simulink model "cyberAttack2"  (R2022b)
settings: Solver=VariableStepAuto  StartTime=0.0  StopTime=10  RelTol=1e-3
values from neighbouring files (symbols this model uses):
  attackTimeDelay = 0.1    [editor.m]
  attackTimeDelay1 = 0.1    [editor.m]
  CC_Kd = 0    [editor.m]
  CC_Ki = 150    [editor.m]
  CC_Kp = 0    [editor.m]
  enableObserver = 1    [editor.m]
  ICapacity_1 = 3    [editor.m]
  ICapacity_2 = 2    [editor.m]
  ILoadFinal = 2    [editor.m]
  ILoadInitial = 3    [editor.m]
  Kd = 4.6e-4    (= 0.00046)    [editor.m]
  Ki = 6.15    [editor.m]
  Kp = 0.1    [editor.m]
  N = 2.56e3    (= 2560)    [editor.m]
  Rij = 0.05    [editor.m]
  Rt = 0.2    [editor.m]
  timeOfAttack = 5    [editor.m]
  timeOfAttack1 = 5    [editor.m]
  tLoadChange = 6    [editor.m]
  Ts = 5e-5    (= 5e-05)    [editor.m]
  Vref = 40    [editor.m]
undefined symbols (not defined in the file or in its folder): Discrete, Time
libraries: fl_lib x54, nesl_utility_internal x30, slpidlib x8, simulink x4, ctrlSharedLib x4, ee_lib x4
(part 2 of 3)

== system cyberAttack2/DGU 1 Observer1 ==
  Vout_3_local : Inport
  It_3_local : Inport  Port=2
  Vt_3 : Inport  Port=3
  Vout_3 : Inport  Port=4
  Vout_4 : Inport  Port=5
  IL : Inport  Port=6
  Disabled : Subsystem  VariantControl=enableObserver == 0
      settings: PortSchema="{\"entries\":[{\"content\":{\"sides\":[{\"content\":{\"connectorIds\":[\"In1\",\"In2\",\"In3\",\"In4\"]},\"type\":\"ConnectorPlacement.EquallySpacedRectSide\",\"uuid\":\"1fcbc3c4-c380-448d-a7a8-357aa057b5ad\"},{\"content\":{\"connectorIds\":[\"Out1\",\"Out2\",\"Out3\"],\"side\":\"RIGHT\"},\"type\":\"ConnectorPlacement.EquallySpacedRectSide\",\"uuid\":\"7cbaad62-7890-4094-8ace-3159eca04825\"},{\"content\":{\"connectorIds\":[\"In5\",\"In6\"],\"side\":\"TOP\"},\"type\":\"ConnectorPlacement.EquallySpacedRectSide\",\"uuid\":\"f6c34017-9df2-4479-96e0-d67eb53c1d2d\"}]},\"type\":\"ConnectorPlacement.EquallySpacedConnector\",\"uuid\":\"f0a4a9b8-ed06-4c65-915f-6b202d377626\"}],\"packageUris\":[\"http://schema.mathworks.com/mf0/Connector/R2020b\"],\"version\":\"1.0\"}"
  Enabled : Subsystem  VariantControl=enableObserver == 1
      settings: PortSchema="{\"entries\":[{\"content\":{\"sides\":[{\"content\":{\"connectorIds\":[\"In1\",\"In2\",\"In3\",\"In4\"]},\"type\":\"ConnectorPlacement.EquallySpacedRectSide\",\"uuid\":\"1fcbc3c4-c380-448d-a7a8-357aa057b5ad\"},{\"content\":{\"connectorIds\":[\"Out1\",\"Out2\",\"Out3\"],\"side\":\"RIGHT\"},\"type\":\"ConnectorPlacement.EquallySpacedRectSide\",\"uuid\":\"7cbaad62-7890-4094-8ace-3159eca04825\"},{\"content\":{\"connectorIds\":[\"In5\",\"In6\"],\"side\":\"TOP\"},\"type\":\"ConnectorPlacement.EquallySpacedRectSide\",\"uuid\":\"f6c34017-9df2-4479-96e0-d67eb53c1d2d\"}]},\"type\":\"ConnectorPlacement.EquallySpacedConnector\",\"uuid\":\"f0a4a9b8-ed06-4c65-915f-6b202d377626\"}],\"packageUris\":[\"http://schema.mathworks.com/mf0/Connector/R2020b\"],\"version\":\"1.0\"}"
  residual_Vout : Outport
  residual_It : Outport  Port=2
  attackDetected : Outport  Port=3

== system cyberAttack2/DGU 2 Observer ==
  Vout_2_local : Inport
  It_2_local : Inport  Port=2
  Vt_2 : Inport  Port=3
  Vout_2 : Inport  Port=4
  Vout_1 : Inport  Port=5
  IL : Inport  Port=6
  Disabled : Subsystem  VariantControl=enableObserver == 0
      settings: PortSchema="{\"entries\":[{\"content\":{\"sides\":[{\"content\":{\"connectorIds\":[\"In1\",\"In2\",\"In3\",\"In4\"]},\"type\":\"ConnectorPlacement.EquallySpacedRectSide\",\"uuid\":\"1fcbc3c4-c380-448d-a7a8-357aa057b5ad\"},{\"content\":{\"connectorIds\":[\"Out1\",\"Out2\",\"Out3\"],\"side\":\"RIGHT\"},\"type\":\"ConnectorPlacement.EquallySpacedRectSide\",\"uuid\":\"7cbaad62-7890-4094-8ace-3159eca04825\"},{\"content\":{\"connectorIds\":[\"In5\",\"In6\"],\"side\":\"TOP\"},\"type\":\"ConnectorPlacement.EquallySpacedRectSide\",\"uuid\":\"f6c34017-9df2-4479-96e0-d67eb53c1d2d\"}]},\"type\":\"ConnectorPlacement.EquallySpacedConnector\",\"uuid\":\"f0a4a9b8-ed06-4c65-915f-6b202d377626\"}],\"packageUris\":[\"http://schema.mathworks.com/mf0/Connector/R2020b\"],\"version\":\"1.0\"}"
  Enabled : Subsystem  VariantControl=enableObserver == 1
      settings: PortSchema="{\"entries\":[{\"content\":{\"sides\":[{\"content\":{\"connectorIds\":[\"In1\",\"In2\",\"In3\",\"In4\"]},\"type\":\"ConnectorPlacement.EquallySpacedRectSide\",\"uuid\":\"1fcbc3c4-c380-448d-a7a8-357aa057b5ad\"},{\"content\":{\"connectorIds\":[\"Out1\",\"Out2\",\"Out3\"],\"side\":\"RIGHT\"},\"type\":\"ConnectorPlacement.EquallySpacedRectSide\",\"uuid\":\"7cbaad62-7890-4094-8ace-3159eca04825\"},{\"content\":{\"connectorIds\":[\"In5\",\"In6\"],\"side\":\"TOP\"},\"type\":\"ConnectorPlacement.EquallySpacedRectSide\",\"uuid\":\"f6c34017-9df2-4479-96e0-d67eb53c1d2d\"}]},\"type\":\"ConnectorPlacement.EquallySpacedConnector\",\"uuid\":\"f0a4a9b8-ed06-4c65-915f-6b202d377626\"}],\"packageUris\":[\"http://schema.mathworks.com/mf0/Connector/R2020b\"],\"version\":\"1.0\"}"
  residual_Vout : Outport
  residual_It : Outport  Port=2
  attackDetected : Outport  Port=3

== system cyberAttack2/DGU 2 Observer1 ==
  Vout_4_local : Inport
  It_4_local : Inport  Port=2
  Vt_4 : Inport  Port=3
  Vout_4 : Inport  Port=4
  Vout_3 : Inport  Port=5
  IL : Inport  Port=6
  Disabled : Subsystem  VariantControl=enableObserver == 0
      settings: PortSchema="{\"entries\":[{\"content\":{\"sides\":[{\"content\":{\"connectorIds\":[\"In1\",\"In2\",\"In3\",\"In4\"]},\"type\":\"ConnectorPlacement.EquallySpacedRectSide\",\"uuid\":\"1fcbc3c4-c380-448d-a7a8-357aa057b5ad\"},{\"content\":{\"connectorIds\":[\"Out1\",\"Out2\",\"Out3\"],\"side\":\"RIGHT\"},\"type\":\"ConnectorPlacement.EquallySpacedRectSide\",\"uuid\":\"7cbaad62-7890-4094-8ace-3159eca04825\"},{\"content\":{\"connectorIds\":[\"In5\",\"In6\"],\"side\":\"TOP\"},\"type\":\"ConnectorPlacement.EquallySpacedRectSide\",\"uuid\":\"f6c34017-9df2-4479-96e0-d67eb53c1d2d\"}]},\"type\":\"ConnectorPlacement.EquallySpacedConnector\",\"uuid\":\"f0a4a9b8-ed06-4c65-915f-6b202d377626\"}],\"packageUris\":[\"http://schema.mathworks.com/mf0/Connector/R2020b\"],\"version\":\"1.0\"}"
  Enabled : Subsystem  VariantControl=enableObserver == 1
      settings: PortSchema="{\"entries\":[{\"content\":{\"sides\":[{\"content\":{\"connectorIds\":[\"In1\",\"In2\",\"In3\",\"In4\"]},\"type\":\"ConnectorPlacement.EquallySpacedRectSide\",\"uuid\":\"1fcbc3c4-c380-448d-a7a8-357aa057b5ad\"},{\"content\":{\"connectorIds\":[\"Out1\",\"Out2\",\"Out3\"],\"side\":\"RIGHT\"},\"type\":\"ConnectorPlacement.EquallySpacedRectSide\",\"uuid\":\"7cbaad62-7890-4094-8ace-3159eca04825\"},{\"content\":{\"connectorIds\":[\"In5\",\"In6\"],\"side\":\"TOP\"},\"type\":\"ConnectorPlacement.EquallySpacedRectSide\",\"uuid\":\"f6c34017-9df2-4479-96e0-d67eb53c1d2d\"}]},\"type\":\"ConnectorPlacement.EquallySpacedConnector\",\"uuid\":\"f0a4a9b8-ed06-4c65-915f-6b202d377626\"}],\"packageUris\":[\"http://schema.mathworks.com/mf0/Connector/R2020b\"],\"version\":\"1.0\"}"
  residual_Vout : Outport
  residual_It : Outport  Port=2
  attackDetected : Outport  Port=3

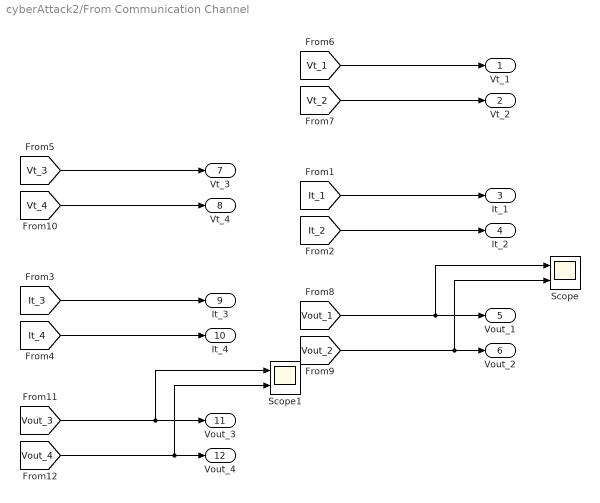
== system cyberAttack2/From Communication Channel ==
  Scope : Scope  NumInputPorts=2
  Scope1 : Scope  NumInputPorts=2
  Vt_1 : Outport
  Vt_2 : Outport  Port=2
  It_1 : Outport  Port=3
  It_2 : Outport  Port=4
  Vout_1 : Outport  Port=5
  Vout_2 : Outport  Port=6
  Vt_3 : Outport  Port=7
  Vt_4 : Outport  Port=8
  It_3 : Outport  Port=9
  It_4 : Outport  Port=10
  Vout_3 : Outport  Port=11
  Vout_4 : Outport  Port=12
  wires:
  [Vout_2] -> Scope/2, Vout_2/1
  [Vt_1] -> Vt_1/1
  [It_1] -> It_1/1
  [Vout_1] -> Scope/1, Vout_1/1
  [Vt_2] -> Vt_2/1
  [It_2] -> It_2/1
  [Vout_4] -> Scope1/2, Vout_4/1
  [Vout_3] -> Scope1/1, Vout_3/1
  [Vt_3] -> Vt_3/1
  [Vt_4] -> Vt_4/1
  [It_3] -> It_3/1
  [It_4] -> It_4/1

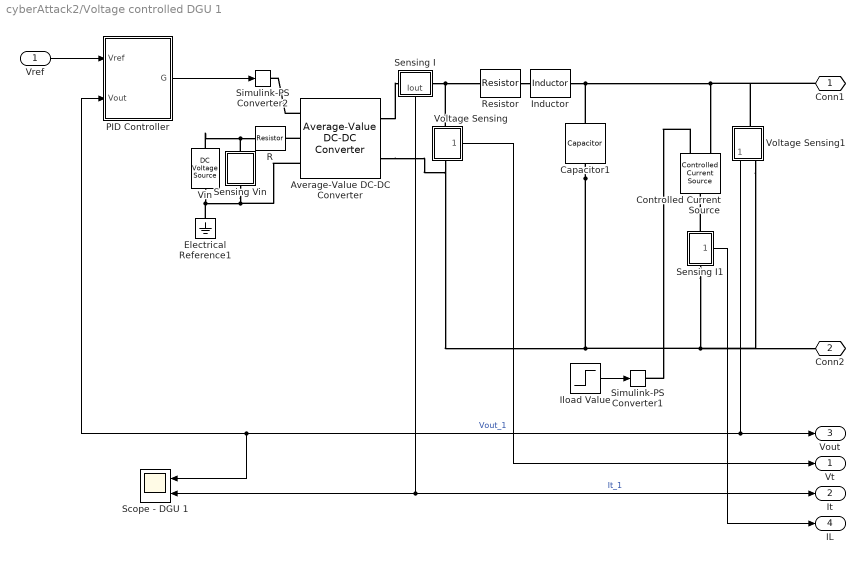
== system cyberAttack2/Voltage controlled DGU 1 ==
  Vref : Inport
  Average-Value DC-DC Converter : ee_lib/Semiconductors & Converters/Converters/Average-Value DC-DC Converter  control_option=ee.enum.converters.controlinput.dutycycle  converter_type=ee.enum.converters.dcdctype.buck  efficiency_option=ee.enum.converters.efficiency.constant  efficiency_fixed=100  i_vec=[0, 2, 5] A  efficiency_vec=[90, 95, 98]
      settings: InternalSimscapePortConfiguration="{\"Bottom\":[],\"Left\":[{\"id\":\"DutyCycle\",\"label\":\"DutyCycle\",\"type\":\"input\"},{\"id\":\"p1\",\"label\":\"1+\",\"type\":\"foundation.electrical.electrical\"},{\"id\":\"n1\",\"label\":\"1-\",\"type\":\"foundation.electrical.electrical\"}],\"Right\":[{\"id\":\"p2\",\"label\":\"2+\",\"type\":\"foundation.electrical.electrical\"},{\"id\":\"n2\",\"label\":\"2-\",\"type\":\"foundation.electrical.electrical\"}],\"Top\":[]}"
  Capacitor1 : fl_lib/Electrical/Electrical Elements/Capacitor  c=Ct F  r=1e-6 Ohm  g=0 1/Ohm  i_specify=off  i_priority=None  i=0 A  i_nominal_specify=off  i_nominal_unit=A  i_nominal_value=1  v_specify=on  v_priority=None  v=80 V  v_nominal_specify=off  v_nominal_unit=V  v_nominal_value=1  vc_specify=off  vc_priority=High  vc=0 V  vc_nominal_specify=off  vc_nominal_unit=V  vc_nominal_value=1
  Controlled Current Source : fl_lib/Electrical/Electrical Sources/Controlled Current Source
  Electrical Reference1 : fl_lib/Electrical/Electrical Elements/Electrical Reference
  Iload Value : Step  Time=tLoadChange  Before=ILoadInitial  After=ILoadFinal  SampleTime=Ts  VectorParams1D=off
  Inductor : fl_lib/Electrical/Electrical Elements/Inductor  l=Lt H  r=0 Ohm  g=1e-9 1/Ohm  i_specify=off  i_priority=None  i=0 A  i_nominal_specify=off  i_nominal_unit=A  i_nominal_value=1  v_specify=off  v_priority=None  v=0 V  v_nominal_specify=off  v_nominal_unit=V  v_nominal_value=1  i_L_specify=off  i_L_priority=High  i_L=0 A  i_L_nominal_specify=off  i_L_nominal_unit=A  i_L_nominal_value=1
  PID Controller : Subsystem  VariantControl=PID Controller
  R : fl_lib/Electrical/Electrical Elements/Resistor  R=0.001 Ohm  i_specify=off  i_priority=None  i=0 A  i_nominal_specify=off  i_nominal_unit=A  i_nominal_value=1  v_specify=off  v_priority=None  v=0 V  v_nominal_specify=off  v_nominal_unit=V  v_nominal_value=1
  Resistor : fl_lib/Electrical/Electrical Elements/Resistor  R=Rt Ohm  i_specify=off  i_priority=None  i=0 A  i_nominal_specify=off  i_nominal_unit=A  i_nominal_value=1  v_specify=off  v_priority=None  v=0 V  v_nominal_specify=off  v_nominal_unit=V  v_nominal_value=1
  Scope - DGU 1 : Scope  NumInputPorts=2
  Sensing Vin : Subsystem
      mask Display:
      | disp('V')
      | port_label('Lconn',1,'+')
      | port_label('Rconn',1,'-')
  Sensing I : Subsystem
      settings: PortSchema="{\"entries\":[{\"content\":{\"sides\":[{\"content\":{\"connectorIds\":[\"LConn1\"]},\"type\":\"ConnectorPlacement.EquallySpacedRectSide\",\"uuid\":\"8998040f-d19b-40f6-852f-9dc0afd5a871\"},{\"content\":{\"connectorIds\":[\"RConn1\"],\"side\":\"RIGHT\"},\"type\":\"ConnectorPlacement.EquallySpacedRectSide\",\"uuid\":\"65494d6e-d653-4050-90f0-55ab431a5ea5\"},{\"content\":{\"connectorIds\":[],\"side\":\"TOP\"},\"type\":\"ConnectorPlacement.EquallySpacedRectSide\",\"uuid\":\"2b796c8d-afa9-4f67-a302-9fd74e5c5a87\"},{\"content\":{\"connectorIds\":[\"Out1\"],\"side\":\"BOTTOM\"},\"type\":\"ConnectorPlacement.EquallySpacedRectSide\",\"uuid\":\"a59db07b-fad7-4423-9f0d-248c8e243318\"}]},\"type\":\"ConnectorPlacement.EquallySpacedConnector\",\"uuid\":\"55bdfac7-fde1-4547-95b0-f675ec2b07db\"}],\"packageUris\":[\"http://schema.mathworks.com/mf0/Connector/R2020b\"],\"version\":\"1.0\"}"
      mask Display:
      | disp('I')
      | port_label('Lconn',1,'+')
      | port_label('Rconn',1,'-')
  Sensing I1 : Subsystem
      settings: PortSchema="{\"entries\":[{\"content\":{\"sides\":[{\"content\":{\"connectorIds\":[\"LConn1\"]},\"type\":\"ConnectorPlacement.EquallySpacedRectSide\",\"uuid\":\"8998040f-d19b-40f6-852f-9dc0afd5a871\"},{\"content\":{\"connectorIds\":[\"RConn1\"],\"side\":\"RIGHT\"},\"type\":\"ConnectorPlacement.EquallySpacedRectSide\",\"uuid\":\"65494d6e-d653-4050-90f0-55ab431a5ea5\"},{\"content\":{\"connectorIds\":[\"Out1\"],\"side\":\"TOP\"},\"type\":\"ConnectorPlacement.EquallySpacedRectSide\",\"uuid\":\"2b796c8d-afa9-4f67-a302-9fd74e5c5a87\"},{\"content\":{\"connectorIds\":[],\"side\":\"BOTTOM\"},\"type\":\"ConnectorPlacement.EquallySpacedRectSide\",\"uuid\":\"a59db07b-fad7-4423-9f0d-248c8e243318\"}]},\"type\":\"ConnectorPlacement.EquallySpacedConnector\",\"uuid\":\"55bdfac7-fde1-4547-95b0-f675ec2b07db\"}],\"packageUris\":[\"http://schema.mathworks.com/mf0/Connector/R2020b\"],\"version\":\"1.0\"}"
      mask Display:
      | disp('I')
      | port_label('Lconn',1,'+')
      | port_label('Rconn',1,'-')
  Simulink-PS Converter1 : nesl_utility_internal/Simulink-PS Converter  PhysicalDomain=network_engine_domain  SubClassName=ps_input  LeftPortType=input  RightPortType=output  PseudoPeriodic=off  Frequencies=[]  NoiseDistribution=none  NoiseParameters=[]  Unit=1  AffineConversion=off  FilteringAndDerivatives=zero  SimscapeFilterOrder=1  InputFilterTimeConstant=0.001  UdotUserProvided=0
  Simulink-PS Converter2 : nesl_utility_internal/Simulink-PS Converter  PhysicalDomain=network_engine_domain  SubClassName=ps_input  LeftPortType=input  RightPortType=output  PseudoPeriodic=off  Frequencies=[]  NoiseDistribution=none  NoiseParameters=[]  Unit=1  AffineConversion=off  FilteringAndDerivatives=provide  SimscapeFilterOrder=1  InputFilterTimeConstant=0.001  UdotUserProvided=0
  Vin : fl_lib/Electrical/Electrical Sources/DC Voltage Source  v0=Vin V
  Voltage Sensing : Subsystem
      settings: PortSchema="{\"entries\":[{\"content\":{\"sides\":[{\"content\":{\"connectorIds\":[\"LConn1\"]},\"type\":\"ConnectorPlacement.EquallySpacedRectSide\",\"uuid\":\"8998040f-d19b-40f6-852f-9dc0afd5a871\"},{\"content\":{\"connectorIds\":[\"RConn1\"],\"side\":\"RIGHT\"},\"type\":\"ConnectorPlacement.EquallySpacedRectSide\",\"uuid\":\"65494d6e-d653-4050-90f0-55ab431a5ea5\"},{\"content\":{\"connectorIds\":[],\"side\":\"TOP\"},\"type\":\"ConnectorPlacement.EquallySpacedRectSide\",\"uuid\":\"2b796c8d-afa9-4f67-a302-9fd74e5c5a87\"},{\"content\":{\"connectorIds\":[\"Out1\"],\"side\":\"BOTTOM\"},\"type\":\"ConnectorPlacement.EquallySpacedRectSide\",\"uuid\":\"603bcbba-3a86-43b0-b8d3-5ff10845ef5f\"}]},\"type\":\"ConnectorPlacement.EquallySpacedConnector\",\"uuid\":\"55bdfac7-fde1-4547-95b0-f675ec2b07db\"}],\"packageUris\":[\"http://schema.mathworks.com/mf0/Connector/R2020b\"],\"version\":\"1.0\"}"
      mask Display:
      | disp('V')
      | port_label('Lconn',1,'+')
      | port_label('Rconn',1,'-')
  Voltage Sensing1 : Subsystem
      mask Display:
      | disp('V')
      | port_label('Lconn',1,'+')
      | port_label('Rconn',1,'-')
  Conn1 : PMIOPort  Side=Right
  Conn2 : PMIOPort  Port=2  Side=Right
  Vt : Outport
  It : Outport  Port=2
  Vout : Outport  Port=3
  IL : Outport  Port=4
  wires:
  PID Controller/1(G) -> Simulink-PS Converter2/1
  Voltage Sensing1/1(Vout) -> Scope - DGU 1/1, PID Controller/2(Vout), Vout/1  "Vout_1"
  Iload Value/1 -> Simulink-PS Converter1/1
  Vref/1 -> PID Controller/1(Vref)
  Sensing I/1(Iout) -> Scope - DGU 1/2, It/1  "It_1"
  Voltage Sensing/1(Out1) -> Vt/1
  Sensing I1/1(Iout) -> IL/1
  connections:
  Capacitor1/LConn1 -- Inductor/RConn1 -- Conn1/RConn1 -- Voltage Sensing1/LConn1 -- Controlled Current Source/RConn2
  Vin/LConn1 -- Sensing Vin/LConn1 -- R/LConn1
  Resistor/RConn1 -- Inductor/LConn1
  Voltage Sensing/LConn1 -- Sensing I/RConn1 -- Resistor/LConn1
  Controlled Current Source/RConn1 -- Simulink-PS Converter1/RConn1
  Sensing I1/LConn1 -- Controlled Current Source/LConn1
  Vin/RConn1 -- Average-Value DC-DC Converter/LConn3 -- Sensing Vin/RConn1 -- Electrical Reference1/LConn1
  Capacitor1/RConn1 -- Average-Value DC-DC Converter/RConn2 -- Voltage Sensing/RConn1 -- Voltage Sensing1/RConn1 -- Conn2/RConn1 -- Sensing I1/RConn1
  Average-Value DC-DC Converter/LConn1 -- Simulink-PS Converter2/RConn1
  Average-Value DC-DC Converter/LConn2 -- R/RConn1
  Average-Value DC-DC Converter/RConn1 -- Sensing I/LConn1

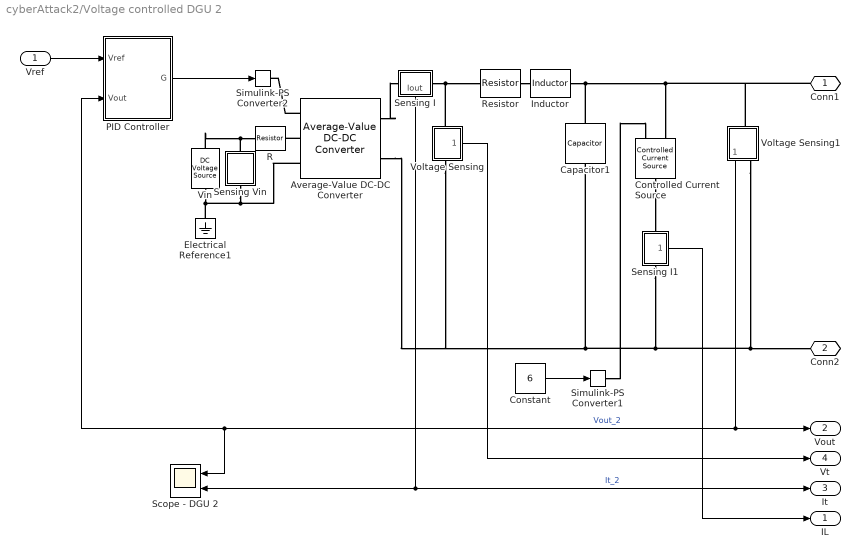
== system cyberAttack2/Voltage controlled DGU 2 ==
  Vref : Inport
  Average-Value DC-DC Converter : ee_lib/Semiconductors & Converters/Converters/Average-Value DC-DC Converter  control_option=ee.enum.converters.controlinput.dutycycle  converter_type=ee.enum.converters.dcdctype.buck  efficiency_option=ee.enum.converters.efficiency.constant  efficiency_fixed=100  i_vec=[0, 2, 5] A  efficiency_vec=[90, 95, 98]
      settings: InternalSimscapePortConfiguration="{\"Bottom\":[],\"Left\":[{\"id\":\"DutyCycle\",\"label\":\"DutyCycle\",\"type\":\"input\"},{\"id\":\"p1\",\"label\":\"1+\",\"type\":\"foundation.electrical.electrical\"},{\"id\":\"n1\",\"label\":\"1-\",\"type\":\"foundation.electrical.electrical\"}],\"Right\":[{\"id\":\"p2\",\"label\":\"2+\",\"type\":\"foundation.electrical.electrical\"},{\"id\":\"n2\",\"label\":\"2-\",\"type\":\"foundation.electrical.electrical\"}],\"Top\":[]}"
  Capacitor1 : fl_lib/Electrical/Electrical Elements/Capacitor  c=Ct F  r=1e-6 Ohm  g=0 1/Ohm  i_specify=off  i_priority=None  i=0 A  i_nominal_specify=off  i_nominal_unit=A  i_nominal_value=1  v_specify=on  v_priority=None  v=80 V  v_nominal_specify=off  v_nominal_unit=V  v_nominal_value=1  vc_specify=off  vc_priority=High  vc=0 V  vc_nominal_specify=off  vc_nominal_unit=V  vc_nominal_value=1
  Constant : Constant  Value=6  SampleTime=Ts
  Controlled Current Source : fl_lib/Electrical/Electrical Sources/Controlled Current Source
  Electrical Reference1 : fl_lib/Electrical/Electrical Elements/Electrical Reference
  Inductor : fl_lib/Electrical/Electrical Elements/Inductor  l=Lt H  r=0 Ohm  g=1e-9 1/Ohm  i_specify=off  i_priority=None  i=0 A  i_nominal_specify=off  i_nominal_unit=A  i_nominal_value=1  v_specify=off  v_priority=None  v=0 V  v_nominal_specify=off  v_nominal_unit=V  v_nominal_value=1  i_L_specify=off  i_L_priority=High  i_L=0 A  i_L_nominal_specify=off  i_L_nominal_unit=A  i_L_nominal_value=1
  PID Controller : Subsystem  VariantControl=PID Controller
  R : fl_lib/Electrical/Electrical Elements/Resistor  R=0.001 Ohm  i_specify=off  i_priority=None  i=0 A  i_nominal_specify=off  i_nominal_unit=A  i_nominal_value=1  v_specify=off  v_priority=None  v=0 V  v_nominal_specify=off  v_nominal_unit=V  v_nominal_value=1
  Resistor : fl_lib/Electrical/Electrical Elements/Resistor  R=Rt Ohm  i_specify=off  i_priority=None  i=0 A  i_nominal_specify=off  i_nominal_unit=A  i_nominal_value=1  v_specify=off  v_priority=None  v=0 V  v_nominal_specify=off  v_nominal_unit=V  v_nominal_value=1
  Scope - DGU 2 : Scope  NumInputPorts=2
  Sensing Vin : Subsystem
      mask Display:
      | disp('V')
      | port_label('Lconn',1,'+')
      | port_label('Rconn',1,'-')
  Sensing I : Subsystem
      settings: PortSchema="{\"entries\":[{\"content\":{\"sides\":[{\"content\":{\"connectorIds\":[\"LConn1\"]},\"type\":\"ConnectorPlacement.EquallySpacedRectSide\",\"uuid\":\"8998040f-d19b-40f6-852f-9dc0afd5a871\"},{\"content\":{\"connectorIds\":[\"RConn1\"],\"side\":\"RIGHT\"},\"type\":\"ConnectorPlacement.EquallySpacedRectSide\",\"uuid\":\"65494d6e-d653-4050-90f0-55ab431a5ea5\"},{\"content\":{\"connectorIds\":[],\"side\":\"TOP\"},\"type\":\"ConnectorPlacement.EquallySpacedRectSide\",\"uuid\":\"2b796c8d-afa9-4f67-a302-9fd74e5c5a87\"},{\"content\":{\"connectorIds\":[\"Out1\"],\"side\":\"BOTTOM\"},\"type\":\"ConnectorPlacement.EquallySpacedRectSide\",\"uuid\":\"a59db07b-fad7-4423-9f0d-248c8e243318\"}]},\"type\":\"ConnectorPlacement.EquallySpacedConnector\",\"uuid\":\"55bdfac7-fde1-4547-95b0-f675ec2b07db\"}],\"packageUris\":[\"http://schema.mathworks.com/mf0/Connector/R2020b\"],\"version\":\"1.0\"}"
      mask Display:
      | disp('I')
      | port_label('Lconn',1,'+')
      | port_label('Rconn',1,'-')
  Sensing I1 : Subsystem
      settings: PortSchema="{\"entries\":[{\"content\":{\"sides\":[{\"content\":{\"connectorIds\":[\"LConn1\"]},\"type\":\"ConnectorPlacement.EquallySpacedRectSide\",\"uuid\":\"8998040f-d19b-40f6-852f-9dc0afd5a871\"},{\"content\":{\"connectorIds\":[\"RConn1\"],\"side\":\"RIGHT\"},\"type\":\"ConnectorPlacement.EquallySpacedRectSide\",\"uuid\":\"65494d6e-d653-4050-90f0-55ab431a5ea5\"},{\"content\":{\"connectorIds\":[\"Out1\"],\"side\":\"TOP\"},\"type\":\"ConnectorPlacement.EquallySpacedRectSide\",\"uuid\":\"2b796c8d-afa9-4f67-a302-9fd74e5c5a87\"},{\"content\":{\"connectorIds\":[],\"side\":\"BOTTOM\"},\"type\":\"ConnectorPlacement.EquallySpacedRectSide\",\"uuid\":\"a59db07b-fad7-4423-9f0d-248c8e243318\"}]},\"type\":\"ConnectorPlacement.EquallySpacedConnector\",\"uuid\":\"55bdfac7-fde1-4547-95b0-f675ec2b07db\"}],\"packageUris\":[\"http://schema.mathworks.com/mf0/Connector/R2020b\"],\"version\":\"1.0\"}"
      mask Display:
      | disp('I')
      | port_label('Lconn',1,'+')
      | port_label('Rconn',1,'-')
  Simulink-PS Converter1 : nesl_utility_internal/Simulink-PS Converter  PhysicalDomain=network_engine_domain  SubClassName=ps_input  LeftPortType=input  RightPortType=output  PseudoPeriodic=off  Frequencies=[]  NoiseDistribution=none  NoiseParameters=[]  Unit=1  AffineConversion=off  FilteringAndDerivatives=zero  SimscapeFilterOrder=1  InputFilterTimeConstant=0.001  UdotUserProvided=0
  Simulink-PS Converter2 : nesl_utility_internal/Simulink-PS Converter  PhysicalDomain=network_engine_domain  SubClassName=ps_input  LeftPortType=input  RightPortType=output  PseudoPeriodic=off  Frequencies=[]  NoiseDistribution=none  NoiseParameters=[]  Unit=1  AffineConversion=off  FilteringAndDerivatives=provide  SimscapeFilterOrder=1  InputFilterTimeConstant=0.001  UdotUserProvided=0
  Vin : fl_lib/Electrical/Electrical Sources/DC Voltage Source  v0=Vin V
  Voltage Sensing : Subsystem
      settings: PortSchema="{\"entries\":[{\"content\":{\"sides\":[{\"content\":{\"connectorIds\":[\"LConn1\"]},\"type\":\"ConnectorPlacement.EquallySpacedRectSide\",\"uuid\":\"8998040f-d19b-40f6-852f-9dc0afd5a871\"},{\"content\":{\"connectorIds\":[\"RConn1\"],\"side\":\"RIGHT\"},\"type\":\"ConnectorPlacement.EquallySpacedRectSide\",\"uuid\":\"65494d6e-d653-4050-90f0-55ab431a5ea5\"},{\"content\":{\"connectorIds\":[],\"side\":\"TOP\"},\"type\":\"ConnectorPlacement.EquallySpacedRectSide\",\"uuid\":\"2b796c8d-afa9-4f67-a302-9fd74e5c5a87\"},{\"content\":{\"connectorIds\":[\"Out1\"],\"side\":\"BOTTOM\"},\"type\":\"ConnectorPlacement.EquallySpacedRectSide\",\"uuid\":\"603bcbba-3a86-43b0-b8d3-5ff10845ef5f\"}]},\"type\":\"ConnectorPlacement.EquallySpacedConnector\",\"uuid\":\"55bdfac7-fde1-4547-95b0-f675ec2b07db\"}],\"packageUris\":[\"http://schema.mathworks.com/mf0/Connector/R2020b\"],\"version\":\"1.0\"}"
      mask Display:
      | disp('V')
      | port_label('Lconn',1,'+')
      | port_label('Rconn',1,'-')
  Voltage Sensing1 : Subsystem
      mask Display:
      | disp('V')
      | port_label('Lconn',1,'+')
      | port_label('Rconn',1,'-')
  Conn1 : PMIOPort  Side=Right
  Conn2 : PMIOPort  Port=2  Side=Right
  IL : Outport
  Vout : Outport  Port=2
  It : Outport  Port=3
  Vt : Outport  Port=4
  wires:
  PID Controller/1(G) -> Simulink-PS Converter2/1
  Voltage Sensing1/1(Vout) -> PID Controller/2(Vout), Scope - DGU 2/1, Vout/1  "Vout_2"
  Constant/1 -> Simulink-PS Converter1/1
  Vref/1 -> PID Controller/1(Vref)
  Sensing I/1(Iout) -> It/1, Scope - DGU 2/2  "It_2"
  Voltage Sensing/1(Out1) -> Vt/1
  Sensing I1/1(Iout) -> IL/1
  connections:
  Voltage Sensing1/RConn1 -- Conn2/RConn1 -- Sensing I1/RConn1 -- Capacitor1/RConn1 -- Average-Value DC-DC Converter/RConn2 -- Voltage Sensing/RConn1
  Capacitor1/LConn1 -- Inductor/RConn1 -- Conn1/RConn1 -- Voltage Sensing1/LConn1 -- Controlled Current Source/RConn2
  Sensing Vin/RConn1 -- Average-Value DC-DC Converter/LConn3 -- Electrical Reference1/LConn1 -- Vin/RConn1
  Vin/LConn1 -- Sensing Vin/LConn1 -- R/LConn1
  Resistor/RConn1 -- Inductor/LConn1
  Average-Value DC-DC Converter/RConn1 -- Sensing I/LConn1
  Average-Value DC-DC Converter/LConn2 -- R/RConn1
  Average-Value DC-DC Converter/LConn1 -- Simulink-PS Converter2/RConn1
  Voltage Sensing/LConn1 -- Sensing I/RConn1 -- Resistor/LConn1
  Simulink-PS Converter1/RConn1 -- Controlled Current Source/RConn1
  Controlled Current Source/LConn1 -- Sensing I1/LConn1

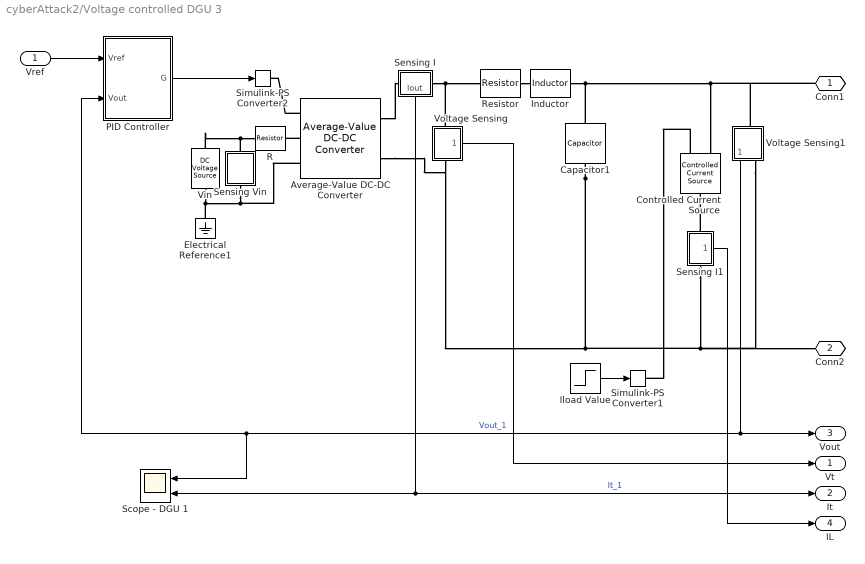
== system cyberAttack2/Voltage controlled DGU 3 ==
  Vref : Inport
  Average-Value DC-DC Converter : ee_lib/Semiconductors & Converters/Converters/Average-Value DC-DC Converter  control_option=ee.enum.converters.controlinput.dutycycle  converter_type=ee.enum.converters.dcdctype.buck  efficiency_option=ee.enum.converters.efficiency.constant  efficiency_fixed=100  i_vec=[0, 2, 5] A  efficiency_vec=[90, 95, 98]
      settings: InternalSimscapePortConfiguration="{\"Bottom\":[],\"Left\":[{\"id\":\"DutyCycle\",\"label\":\"DutyCycle\",\"type\":\"input\"},{\"id\":\"p1\",\"label\":\"1+\",\"type\":\"foundation.electrical.electrical\"},{\"id\":\"n1\",\"label\":\"1-\",\"type\":\"foundation.electrical.electrical\"}],\"Right\":[{\"id\":\"p2\",\"label\":\"2+\",\"type\":\"foundation.electrical.electrical\"},{\"id\":\"n2\",\"label\":\"2-\",\"type\":\"foundation.electrical.electrical\"}],\"Top\":[]}"
  Capacitor1 : fl_lib/Electrical/Electrical Elements/Capacitor  c=Ct F  r=1e-6 Ohm  g=0 1/Ohm  i_specify=off  i_priority=None  i=0 A  i_nominal_specify=off  i_nominal_unit=A  i_nominal_value=1  v_specify=on  v_priority=None  v=80 V  v_nominal_specify=off  v_nominal_unit=V  v_nominal_value=1  vc_specify=off  vc_priority=High  vc=0 V  vc_nominal_specify=off  vc_nominal_unit=V  vc_nominal_value=1
  Controlled Current Source : fl_lib/Electrical/Electrical Sources/Controlled Current Source
  Electrical Reference1 : fl_lib/Electrical/Electrical Elements/Electrical Reference
  Iload Value : Step  Time=tLoadChange  Before=ILoadInitial  After=ILoadFinal  SampleTime=Ts  VectorParams1D=off
  Inductor : fl_lib/Electrical/Electrical Elements/Inductor  l=Lt H  r=0 Ohm  g=1e-9 1/Ohm  i_specify=off  i_priority=None  i=0 A  i_nominal_specify=off  i_nominal_unit=A  i_nominal_value=1  v_specify=off  v_priority=None  v=0 V  v_nominal_specify=off  v_nominal_unit=V  v_nominal_value=1  i_L_specify=off  i_L_priority=High  i_L=0 A  i_L_nominal_specify=off  i_L_nominal_unit=A  i_L_nominal_value=1
  PID Controller : Subsystem  VariantControl=PID Controller
  R : fl_lib/Electrical/Electrical Elements/Resistor  R=0.001 Ohm  i_specify=off  i_priority=None  i=0 A  i_nominal_specify=off  i_nominal_unit=A  i_nominal_value=1  v_specify=off  v_priority=None  v=0 V  v_nominal_specify=off  v_nominal_unit=V  v_nominal_value=1
  Resistor : fl_lib/Electrical/Electrical Elements/Resistor  R=Rt Ohm  i_specify=off  i_priority=None  i=0 A  i_nominal_specify=off  i_nominal_unit=A  i_nominal_value=1  v_specify=off  v_priority=None  v=0 V  v_nominal_specify=off  v_nominal_unit=V  v_nominal_value=1
  Scope - DGU 1 : Scope  NumInputPorts=2
  Sensing Vin : Subsystem
      mask Display:
      | disp('V')
      | port_label('Lconn',1,'+')
      | port_label('Rconn',1,'-')
  Sensing I : Subsystem
      settings: PortSchema="{\"entries\":[{\"content\":{\"sides\":[{\"content\":{\"connectorIds\":[\"LConn1\"]},\"type\":\"ConnectorPlacement.EquallySpacedRectSide\",\"uuid\":\"8998040f-d19b-40f6-852f-9dc0afd5a871\"},{\"content\":{\"connectorIds\":[\"RConn1\"],\"side\":\"RIGHT\"},\"type\":\"ConnectorPlacement.EquallySpacedRectSide\",\"uuid\":\"65494d6e-d653-4050-90f0-55ab431a5ea5\"},{\"content\":{\"connectorIds\":[],\"side\":\"TOP\"},\"type\":\"ConnectorPlacement.EquallySpacedRectSide\",\"uuid\":\"2b796c8d-afa9-4f67-a302-9fd74e5c5a87\"},{\"content\":{\"connectorIds\":[\"Out1\"],\"side\":\"BOTTOM\"},\"type\":\"ConnectorPlacement.EquallySpacedRectSide\",\"uuid\":\"a59db07b-fad7-4423-9f0d-248c8e243318\"}]},\"type\":\"ConnectorPlacement.EquallySpacedConnector\",\"uuid\":\"55bdfac7-fde1-4547-95b0-f675ec2b07db\"}],\"packageUris\":[\"http://schema.mathworks.com/mf0/Connector/R2020b\"],\"version\":\"1.0\"}"
      mask Display:
      | disp('I')
      | port_label('Lconn',1,'+')
      | port_label('Rconn',1,'-')
  Sensing I1 : Subsystem
      settings: PortSchema="{\"entries\":[{\"content\":{\"sides\":[{\"content\":{\"connectorIds\":[\"LConn1\"]},\"type\":\"ConnectorPlacement.EquallySpacedRectSide\",\"uuid\":\"8998040f-d19b-40f6-852f-9dc0afd5a871\"},{\"content\":{\"connectorIds\":[\"RConn1\"],\"side\":\"RIGHT\"},\"type\":\"ConnectorPlacement.EquallySpacedRectSide\",\"uuid\":\"65494d6e-d653-4050-90f0-55ab431a5ea5\"},{\"content\":{\"connectorIds\":[\"Out1\"],\"side\":\"TOP\"},\"type\":\"ConnectorPlacement.EquallySpacedRectSide\",\"uuid\":\"2b796c8d-afa9-4f67-a302-9fd74e5c5a87\"},{\"content\":{\"connectorIds\":[],\"side\":\"BOTTOM\"},\"type\":\"ConnectorPlacement.EquallySpacedRectSide\",\"uuid\":\"a59db07b-fad7-4423-9f0d-248c8e243318\"}]},\"type\":\"ConnectorPlacement.EquallySpacedConnector\",\"uuid\":\"55bdfac7-fde1-4547-95b0-f675ec2b07db\"}],\"packageUris\":[\"http://schema.mathworks.com/mf0/Connector/R2020b\"],\"version\":\"1.0\"}"
      mask Display:
      | disp('I')
      | port_label('Lconn',1,'+')
      | port_label('Rconn',1,'-')
  Simulink-PS Converter1 : nesl_utility_internal/Simulink-PS Converter  PhysicalDomain=network_engine_domain  SubClassName=ps_input  LeftPortType=input  RightPortType=output  PseudoPeriodic=off  Frequencies=[]  NoiseDistribution=none  NoiseParameters=[]  Unit=1  AffineConversion=off  FilteringAndDerivatives=zero  SimscapeFilterOrder=1  InputFilterTimeConstant=0.001  UdotUserProvided=0
  Simulink-PS Converter2 : nesl_utility_internal/Simulink-PS Converter  PhysicalDomain=network_engine_domain  SubClassName=ps_input  LeftPortType=input  RightPortType=output  PseudoPeriodic=off  Frequencies=[]  NoiseDistribution=none  NoiseParameters=[]  Unit=1  AffineConversion=off  FilteringAndDerivatives=provide  SimscapeFilterOrder=1  InputFilterTimeConstant=0.001  UdotUserProvided=0
  Vin : fl_lib/Electrical/Electrical Sources/DC Voltage Source  v0=Vin V
  Voltage Sensing : Subsystem
      settings: PortSchema="{\"entries\":[{\"content\":{\"sides\":[{\"content\":{\"connectorIds\":[\"LConn1\"]},\"type\":\"ConnectorPlacement.EquallySpacedRectSide\",\"uuid\":\"8998040f-d19b-40f6-852f-9dc0afd5a871\"},{\"content\":{\"connectorIds\":[\"RConn1\"],\"side\":\"RIGHT\"},\"type\":\"ConnectorPlacement.EquallySpacedRectSide\",\"uuid\":\"65494d6e-d653-4050-90f0-55ab431a5ea5\"},{\"content\":{\"connectorIds\":[],\"side\":\"TOP\"},\"type\":\"ConnectorPlacement.EquallySpacedRectSide\",\"uuid\":\"2b796c8d-afa9-4f67-a302-9fd74e5c5a87\"},{\"content\":{\"connectorIds\":[\"Out1\"],\"side\":\"BOTTOM\"},\"type\":\"ConnectorPlacement.EquallySpacedRectSide\",\"uuid\":\"603bcbba-3a86-43b0-b8d3-5ff10845ef5f\"}]},\"type\":\"ConnectorPlacement.EquallySpacedConnector\",\"uuid\":\"55bdfac7-fde1-4547-95b0-f675ec2b07db\"}],\"packageUris\":[\"http://schema.mathworks.com/mf0/Connector/R2020b\"],\"version\":\"1.0\"}"
      mask Display:
      | disp('V')
      | port_label('Lconn',1,'+')
      | port_label('Rconn',1,'-')
  Voltage Sensing1 : Subsystem
      mask Display:
      | disp('V')
      | port_label('Lconn',1,'+')
      | port_label('Rconn',1,'-')
  Conn1 : PMIOPort  Side=Right
  Conn2 : PMIOPort  Port=2  Side=Right
  Vt : Outport
  It : Outport  Port=2
  Vout : Outport  Port=3
  IL : Outport  Port=4
  wires:
  PID Controller/1(G) -> Simulink-PS Converter2/1
  Voltage Sensing1/1(Vout) -> Scope - DGU 1/1, PID Controller/2(Vout), Vout/1  "Vout_1"
  Iload Value/1 -> Simulink-PS Converter1/1
  Vref/1 -> PID Controller/1(Vref)
  Sensing I/1(Iout) -> Scope - DGU 1/2, It/1  "It_1"
  Voltage Sensing/1(Out1) -> Vt/1
  Sensing I1/1(Iout) -> IL/1
  connections:
  Capacitor1/LConn1 -- Inductor/RConn1 -- Conn1/RConn1 -- Voltage Sensing1/LConn1 -- Controlled Current Source/RConn2
  Vin/LConn1 -- Sensing Vin/LConn1 -- R/LConn1
  Resistor/RConn1 -- Inductor/LConn1
  Voltage Sensing/LConn1 -- Sensing I/RConn1 -- Resistor/LConn1
  Controlled Current Source/RConn1 -- Simulink-PS Converter1/RConn1
  Sensing I1/LConn1 -- Controlled Current Source/LConn1
  Vin/RConn1 -- Average-Value DC-DC Converter/LConn3 -- Sensing Vin/RConn1 -- Electrical Reference1/LConn1
  Capacitor1/RConn1 -- Average-Value DC-DC Converter/RConn2 -- Voltage Sensing/RConn1 -- Voltage Sensing1/RConn1 -- Conn2/RConn1 -- Sensing I1/RConn1
  Average-Value DC-DC Converter/LConn1 -- Simulink-PS Converter2/RConn1
  Average-Value DC-DC Converter/LConn2 -- R/RConn1
  Average-Value DC-DC Converter/RConn1 -- Sensing I/LConn1

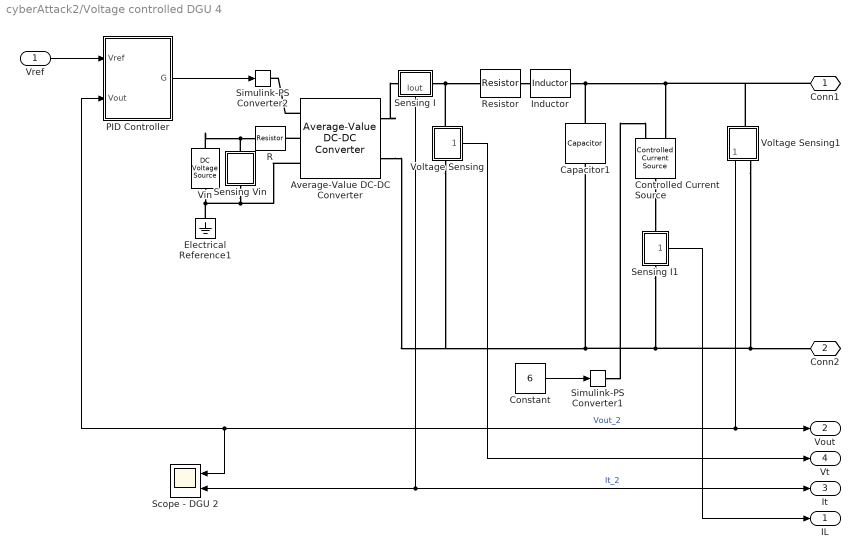
== system cyberAttack2/Voltage controlled DGU 4 ==
  Vref : Inport
  Average-Value DC-DC Converter : ee_lib/Semiconductors & Converters/Converters/Average-Value DC-DC Converter  control_option=ee.enum.converters.controlinput.dutycycle  converter_type=ee.enum.converters.dcdctype.buck  efficiency_option=ee.enum.converters.efficiency.constant  efficiency_fixed=100  i_vec=[0, 2, 5] A  efficiency_vec=[90, 95, 98]
      settings: InternalSimscapePortConfiguration="{\"Bottom\":[],\"Left\":[{\"id\":\"DutyCycle\",\"label\":\"DutyCycle\",\"type\":\"input\"},{\"id\":\"p1\",\"label\":\"1+\",\"type\":\"foundation.electrical.electrical\"},{\"id\":\"n1\",\"label\":\"1-\",\"type\":\"foundation.electrical.electrical\"}],\"Right\":[{\"id\":\"p2\",\"label\":\"2+\",\"type\":\"foundation.electrical.electrical\"},{\"id\":\"n2\",\"label\":\"2-\",\"type\":\"foundation.electrical.electrical\"}],\"Top\":[]}"
  Capacitor1 : fl_lib/Electrical/Electrical Elements/Capacitor  c=Ct F  r=1e-6 Ohm  g=0 1/Ohm  i_specify=off  i_priority=None  i=0 A  i_nominal_specify=off  i_nominal_unit=A  i_nominal_value=1  v_specify=on  v_priority=None  v=80 V  v_nominal_specify=off  v_nominal_unit=V  v_nominal_value=1  vc_specify=off  vc_priority=High  vc=0 V  vc_nominal_specify=off  vc_nominal_unit=V  vc_nominal_value=1
  Constant : Constant  Value=6  SampleTime=Ts
  Controlled Current Source : fl_lib/Electrical/Electrical Sources/Controlled Current Source
  Electrical Reference1 : fl_lib/Electrical/Electrical Elements/Electrical Reference
  Inductor : fl_lib/Electrical/Electrical Elements/Inductor  l=Lt H  r=0 Ohm  g=1e-9 1/Ohm  i_specify=off  i_priority=None  i=0 A  i_nominal_specify=off  i_nominal_unit=A  i_nominal_value=1  v_specify=off  v_priority=None  v=0 V  v_nominal_specify=off  v_nominal_unit=V  v_nominal_value=1  i_L_specify=off  i_L_priority=High  i_L=0 A  i_L_nominal_specify=off  i_L_nominal_unit=A  i_L_nominal_value=1
  PID Controller : Subsystem  VariantControl=PID Controller
  R : fl_lib/Electrical/Electrical Elements/Resistor  R=0.001 Ohm  i_specify=off  i_priority=None  i=0 A  i_nominal_specify=off  i_nominal_unit=A  i_nominal_value=1  v_specify=off  v_priority=None  v=0 V  v_nominal_specify=off  v_nominal_unit=V  v_nominal_value=1
  Resistor : fl_lib/Electrical/Electrical Elements/Resistor  R=Rt Ohm  i_specify=off  i_priority=None  i=0 A  i_nominal_specify=off  i_nominal_unit=A  i_nominal_value=1  v_specify=off  v_priority=None  v=0 V  v_nominal_specify=off  v_nominal_unit=V  v_nominal_value=1
  Scope - DGU 2 : Scope  NumInputPorts=2
  Sensing Vin : Subsystem
      mask Display:
      | disp('V')
      | port_label('Lconn',1,'+')
      | port_label('Rconn',1,'-')
  Sensing I : Subsystem
      settings: PortSchema="{\"entries\":[{\"content\":{\"sides\":[{\"content\":{\"connectorIds\":[\"LConn1\"]},\"type\":\"ConnectorPlacement.EquallySpacedRectSide\",\"uuid\":\"8998040f-d19b-40f6-852f-9dc0afd5a871\"},{\"content\":{\"connectorIds\":[\"RConn1\"],\"side\":\"RIGHT\"},\"type\":\"ConnectorPlacement.EquallySpacedRectSide\",\"uuid\":\"65494d6e-d653-4050-90f0-55ab431a5ea5\"},{\"content\":{\"connectorIds\":[],\"side\":\"TOP\"},\"type\":\"ConnectorPlacement.EquallySpacedRectSide\",\"uuid\":\"2b796c8d-afa9-4f67-a302-9fd74e5c5a87\"},{\"content\":{\"connectorIds\":[\"Out1\"],\"side\":\"BOTTOM\"},\"type\":\"ConnectorPlacement.EquallySpacedRectSide\",\"uuid\":\"a59db07b-fad7-4423-9f0d-248c8e243318\"}]},\"type\":\"ConnectorPlacement.EquallySpacedConnector\",\"uuid\":\"55bdfac7-fde1-4547-95b0-f675ec2b07db\"}],\"packageUris\":[\"http://schema.mathworks.com/mf0/Connector/R2020b\"],\"version\":\"1.0\"}"
      mask Display:
      | disp('I')
      | port_label('Lconn',1,'+')
      | port_label('Rconn',1,'-')
  Sensing I1 : Subsystem
      settings: PortSchema="{\"entries\":[{\"content\":{\"sides\":[{\"content\":{\"connectorIds\":[\"LConn1\"]},\"type\":\"ConnectorPlacement.EquallySpacedRectSide\",\"uuid\":\"8998040f-d19b-40f6-852f-9dc0afd5a871\"},{\"content\":{\"connectorIds\":[\"RConn1\"],\"side\":\"RIGHT\"},\"type\":\"ConnectorPlacement.EquallySpacedRectSide\",\"uuid\":\"65494d6e-d653-4050-90f0-55ab431a5ea5\"},{\"content\":{\"connectorIds\":[\"Out1\"],\"side\":\"TOP\"},\"type\":\"ConnectorPlacement.EquallySpacedRectSide\",\"uuid\":\"2b796c8d-afa9-4f67-a302-9fd74e5c5a87\"},{\"content\":{\"connectorIds\":[],\"side\":\"BOTTOM\"},\"type\":\"ConnectorPlacement.EquallySpacedRectSide\",\"uuid\":\"a59db07b-fad7-4423-9f0d-248c8e243318\"}]},\"type\":\"ConnectorPlacement.EquallySpacedConnector\",\"uuid\":\"55bdfac7-fde1-4547-95b0-f675ec2b07db\"}],\"packageUris\":[\"http://schema.mathworks.com/mf0/Connector/R2020b\"],\"version\":\"1.0\"}"
      mask Display:
      | disp('I')
      | port_label('Lconn',1,'+')
      | port_label('Rconn',1,'-')
  Simulink-PS Converter1 : nesl_utility_internal/Simulink-PS Converter  PhysicalDomain=network_engine_domain  SubClassName=ps_input  LeftPortType=input  RightPortType=output  PseudoPeriodic=off  Frequencies=[]  NoiseDistribution=none  NoiseParameters=[]  Unit=1  AffineConversion=off  FilteringAndDerivatives=zero  SimscapeFilterOrder=1  InputFilterTimeConstant=0.001  UdotUserProvided=0
  Simulink-PS Converter2 : nesl_utility_internal/Simulink-PS Converter  PhysicalDomain=network_engine_domain  SubClassName=ps_input  LeftPortType=input  RightPortType=output  PseudoPeriodic=off  Frequencies=[]  NoiseDistribution=none  NoiseParameters=[]  Unit=1  AffineConversion=off  FilteringAndDerivatives=provide  SimscapeFilterOrder=1  InputFilterTimeConstant=0.001  UdotUserProvided=0
  Vin : fl_lib/Electrical/Electrical Sources/DC Voltage Source  v0=Vin V
  Voltage Sensing : Subsystem
      settings: PortSchema="{\"entries\":[{\"content\":{\"sides\":[{\"content\":{\"connectorIds\":[\"LConn1\"]},\"type\":\"ConnectorPlacement.EquallySpacedRectSide\",\"uuid\":\"8998040f-d19b-40f6-852f-9dc0afd5a871\"},{\"content\":{\"connectorIds\":[\"RConn1\"],\"side\":\"RIGHT\"},\"type\":\"ConnectorPlacement.EquallySpacedRectSide\",\"uuid\":\"65494d6e-d653-4050-90f0-55ab431a5ea5\"},{\"content\":{\"connectorIds\":[],\"side\":\"TOP\"},\"type\":\"ConnectorPlacement.EquallySpacedRectSide\",\"uuid\":\"2b796c8d-afa9-4f67-a302-9fd74e5c5a87\"},{\"content\":{\"connectorIds\":[\"Out1\"],\"side\":\"BOTTOM\"},\"type\":\"ConnectorPlacement.EquallySpacedRectSide\",\"uuid\":\"603bcbba-3a86-43b0-b8d3-5ff10845ef5f\"}]},\"type\":\"ConnectorPlacement.EquallySpacedConnector\",\"uuid\":\"55bdfac7-fde1-4547-95b0-f675ec2b07db\"}],\"packageUris\":[\"http://schema.mathworks.com/mf0/Connector/R2020b\"],\"version\":\"1.0\"}"
      mask Display:
      | disp('V')
      | port_label('Lconn',1,'+')
      | port_label('Rconn',1,'-')
  Voltage Sensing1 : Subsystem
      mask Display:
      | disp('V')
      | port_label('Lconn',1,'+')
      | port_label('Rconn',1,'-')
  Conn1 : PMIOPort  Side=Right
  Conn2 : PMIOPort  Port=2  Side=Right
  IL : Outport
  Vout : Outport  Port=2
  It : Outport  Port=3
  Vt : Outport  Port=4
  wires:
  PID Controller/1(G) -> Simulink-PS Converter2/1
  Voltage Sensing1/1(Vout) -> PID Controller/2(Vout), Scope - DGU 2/1, Vout/1  "Vout_2"
  Constant/1 -> Simulink-PS Converter1/1
  Vref/1 -> PID Controller/1(Vref)
  Sensing I/1(Iout) -> It/1, Scope - DGU 2/2  "It_2"
  Voltage Sensing/1(Out1) -> Vt/1
  Sensing I1/1(Iout) -> IL/1
  connections:
  Voltage Sensing1/RConn1 -- Conn2/RConn1 -- Sensing I1/RConn1 -- Capacitor1/RConn1 -- Average-Value DC-DC Converter/RConn2 -- Voltage Sensing/RConn1
  Capacitor1/LConn1 -- Inductor/RConn1 -- Conn1/RConn1 -- Voltage Sensing1/LConn1 -- Controlled Current Source/RConn2
  Sensing Vin/RConn1 -- Average-Value DC-DC Converter/LConn3 -- Electrical Reference1/LConn1 -- Vin/RConn1
  Vin/LConn1 -- Sensing Vin/LConn1 -- R/LConn1
  Resistor/RConn1 -- Inductor/LConn1
  Average-Value DC-DC Converter/RConn1 -- Sensing I/LConn1
  Average-Value DC-DC Converter/LConn2 -- R/RConn1
  Average-Value DC-DC Converter/LConn1 -- Simulink-PS Converter2/RConn1
  Voltage Sensing/LConn1 -- Sensing I/RConn1 -- Resistor/LConn1
  Simulink-PS Converter1/RConn1 -- Controlled Current Source/RConn1
  Controlled Current Source/LConn1 -- Sensing I1/LConn1

== system cyberAttack2/Add Watermark 1/Disabled ==
  Vt : Inport
  It : Inport  Port=2
  Vout : Inport  Port=3
  Constant : Constant  Value=0  SampleTime=Ts
  Constant1 : Constant  Value=0  SampleTime=Ts
  Constant2 : Constant  Value=0  SampleTime=Ts
  Out2 : Outport
  Out1 : Outport  Port=2
  Out3 : Outport  Port=3
  Out4 : Outport  Port=4
  Out5 : Outport  Port=5
  Out6 : Outport  Port=6
  wires:
  Constant2/1 -> Out6/1
  Vout/1 -> Out3/1
  Constant1/1 -> Out5/1
  It/1 -> Out1/1
  Constant/1 -> Out4/1
  Vt/1 -> Out2/1

== system cyberAttack2/Add Watermark 1/Enabled ==
  Vt : Inport
  It : Inport  Port=2
  Vout : Inport  Port=3
  Add Watermark : Subsystem  mask{MP_SawtoothAmplitude=10, MP_SawtoothFrequency=2}
      mask prompts: MP_SawtoothAmplitude "Sawtooth Amplitude"; MP_SawtoothFrequency "Sawtooth Frequency"
      mask DialogControl ParameterGroupVar Prompt: Sawtooth Watermark Signal
  Add Watermark1 : Subsystem  mask{MP_SawtoothAmplitude=10, MP_SawtoothFrequency=2}
      mask prompts: MP_SawtoothAmplitude "Sawtooth Amplitude"; MP_SawtoothFrequency "Sawtooth Frequency"
      mask DialogControl ParameterGroupVar Prompt: Sawtooth Watermark Signal
  Add Watermark2 : Subsystem  mask{MP_SawtoothAmplitude=10, MP_SawtoothFrequency=2}
      mask prompts: MP_SawtoothAmplitude "Sawtooth Amplitude"; MP_SawtoothFrequency "Sawtooth Frequency"
      mask DialogControl ParameterGroupVar Prompt: Sawtooth Watermark Signal
  Scope : Scope
  Out2 : Outport
  Out1 : Outport  Port=2
  Out3 : Outport  Port=3
  Out4 : Outport  Port=4
  Out5 : Outport  Port=5
  Out6 : Outport  Port=6
  wires:
  Vt/1 -> Add Watermark/1(y)
  It/1 -> Add Watermark1/1(y)
  Vout/1 -> Add Watermark2/1(y)
  Add Watermark/1(y_ym) -> Out2/1
  Add Watermark/2(wm) -> Scope/1, Out4/1
  Add Watermark1/1(y_ym) -> Out1/1
  Add Watermark1/2(wm) -> Out5/1
  Add Watermark2/1(y_ym) -> Out3/1
  Add Watermark2/2(wm) -> Out6/1

== system cyberAttack2/Add Watermark 2/Disabled ==
  Vt : Inport
  It : Inport  Port=2
  Vout : Inport  Port=3
  Constant : Constant  Value=0  SampleTime=Ts
  Constant1 : Constant  Value=0  SampleTime=Ts
  Constant2 : Constant  Value=0  SampleTime=Ts
  Out2 : Outport
  Out1 : Outport  Port=2
  Out3 : Outport  Port=3
  Out4 : Outport  Port=4
  Out5 : Outport  Port=5
  Out6 : Outport  Port=6
  wires:
  Constant2/1 -> Out6/1
  Vout/1 -> Out3/1
  Constant1/1 -> Out5/1
  It/1 -> Out1/1
  Constant/1 -> Out4/1
  Vt/1 -> Out2/1

== system cyberAttack2/Add Watermark 2/Enabled ==
  Vt : Inport
  It : Inport  Port=2
  Vout : Inport  Port=3
  Add Watermark : Subsystem  mask{MP_SawtoothAmplitude=10, MP_SawtoothFrequency=2}
      mask prompts: MP_SawtoothAmplitude "Sawtooth Amplitude"; MP_SawtoothFrequency "Sawtooth Frequency"
      mask DialogControl ParameterGroupVar Prompt: Sawtooth Watermark Signal
  Add Watermark1 : Subsystem  mask{MP_SawtoothAmplitude=10, MP_SawtoothFrequency=2}
      mask prompts: MP_SawtoothAmplitude "Sawtooth Amplitude"; MP_SawtoothFrequency "Sawtooth Frequency"
      mask DialogControl ParameterGroupVar Prompt: Sawtooth Watermark Signal
  Add Watermark2 : Subsystem  mask{MP_SawtoothAmplitude=10, MP_SawtoothFrequency=2}
      mask prompts: MP_SawtoothAmplitude "Sawtooth Amplitude"; MP_SawtoothFrequency "Sawtooth Frequency"
      mask DialogControl ParameterGroupVar Prompt: Sawtooth Watermark Signal
  Out2 : Outport
  Out1 : Outport  Port=2
  Out3 : Outport  Port=3
  Out4 : Outport  Port=4
  Out5 : Outport  Port=5
  Out6 : Outport  Port=6
  wires:
  Vt/1 -> Add Watermark/1(y)
  It/1 -> Add Watermark1/1(y)
  Vout/1 -> Add Watermark2/1(y)
  Add Watermark/1(y_ym) -> Out2/1
  Add Watermark/2(wm) -> Out4/1
  Add Watermark1/1(y_ym) -> Out1/1
  Add Watermark1/2(wm) -> Out5/1
  Add Watermark2/1(y_ym) -> Out3/1
  Add Watermark2/2(wm) -> Out6/1

== system cyberAttack2/Add Watermark 3/Disabled ==
  Vt : Inport
  It : Inport  Port=2
  Vout : Inport  Port=3
  Constant : Constant  Value=0  SampleTime=Ts
  Constant1 : Constant  Value=0  SampleTime=Ts
  Constant2 : Constant  Value=0  SampleTime=Ts
  Out2 : Outport
  Out1 : Outport  Port=2
  Out3 : Outport  Port=3
  Out4 : Outport  Port=4
  Out5 : Outport  Port=5
  Out6 : Outport  Port=6
  wires:
  Constant2/1 -> Out6/1
  Vout/1 -> Out3/1
  Constant1/1 -> Out5/1
  It/1 -> Out1/1
  Constant/1 -> Out4/1
  Vt/1 -> Out2/1

== system cyberAttack2/Add Watermark 3/Enabled ==
  Vt : Inport
  It : Inport  Port=2
  Vout : Inport  Port=3
  Add Watermark : Subsystem  mask{MP_SawtoothAmplitude=10, MP_SawtoothFrequency=2}
      mask prompts: MP_SawtoothAmplitude "Sawtooth Amplitude"; MP_SawtoothFrequency "Sawtooth Frequency"
      mask DialogControl ParameterGroupVar Prompt: Sawtooth Watermark Signal
  Add Watermark1 : Subsystem  mask{MP_SawtoothAmplitude=10, MP_SawtoothFrequency=2}
      mask prompts: MP_SawtoothAmplitude "Sawtooth Amplitude"; MP_SawtoothFrequency "Sawtooth Frequency"
      mask DialogControl ParameterGroupVar Prompt: Sawtooth Watermark Signal
  Add Watermark2 : Subsystem  mask{MP_SawtoothAmplitude=10, MP_SawtoothFrequency=2}
      mask prompts: MP_SawtoothAmplitude "Sawtooth Amplitude"; MP_SawtoothFrequency "Sawtooth Frequency"
      mask DialogControl ParameterGroupVar Prompt: Sawtooth Watermark Signal
  Scope : Scope
  Out2 : Outport
  Out1 : Outport  Port=2
  Out3 : Outport  Port=3
  Out4 : Outport  Port=4
  Out5 : Outport  Port=5
  Out6 : Outport  Port=6
  wires:
  Vt/1 -> Add Watermark/1(y)
  It/1 -> Add Watermark1/1(y)
  Vout/1 -> Add Watermark2/1(y)
  Add Watermark/1(y_ym) -> Out2/1
  Add Watermark/2(wm) -> Scope/1, Out4/1
  Add Watermark1/1(y_ym) -> Out1/1
  Add Watermark1/2(wm) -> Out5/1
  Add Watermark2/1(y_ym) -> Out3/1
  Add Watermark2/2(wm) -> Out6/1

== system cyberAttack2/Add Watermark 4/Disabled ==
  Vt : Inport
  It : Inport  Port=2
  Vout : Inport  Port=3
  Constant : Constant  Value=0  SampleTime=Ts
  Constant1 : Constant  Value=0  SampleTime=Ts
  Constant2 : Constant  Value=0  SampleTime=Ts
  Out2 : Outport
  Out1 : Outport  Port=2
  Out3 : Outport  Port=3
  Out4 : Outport  Port=4
  Out5 : Outport  Port=5
  Out6 : Outport  Port=6
  wires:
  Constant2/1 -> Out6/1
  Vout/1 -> Out3/1
  Constant1/1 -> Out5/1
  It/1 -> Out1/1
  Constant/1 -> Out4/1
  Vt/1 -> Out2/1

== system cyberAttack2/Add Watermark 4/Enabled ==
  Vt : Inport
  It : Inport  Port=2
  Vout : Inport  Port=3
  Add Watermark : Subsystem  mask{MP_SawtoothAmplitude=10, MP_SawtoothFrequency=2}
      mask prompts: MP_SawtoothAmplitude "Sawtooth Amplitude"; MP_SawtoothFrequency "Sawtooth Frequency"
      mask DialogControl ParameterGroupVar Prompt: Sawtooth Watermark Signal
  Add Watermark1 : Subsystem  mask{MP_SawtoothAmplitude=10, MP_SawtoothFrequency=2}
      mask prompts: MP_SawtoothAmplitude "Sawtooth Amplitude"; MP_SawtoothFrequency "Sawtooth Frequency"
      mask DialogControl ParameterGroupVar Prompt: Sawtooth Watermark Signal
  Add Watermark2 : Subsystem  mask{MP_SawtoothAmplitude=10, MP_SawtoothFrequency=2}
      mask prompts: MP_SawtoothAmplitude "Sawtooth Amplitude"; MP_SawtoothFrequency "Sawtooth Frequency"
      mask DialogControl ParameterGroupVar Prompt: Sawtooth Watermark Signal
  Out2 : Outport
  Out1 : Outport  Port=2
  Out3 : Outport  Port=3
  Out4 : Outport  Port=4
  Out5 : Outport  Port=5
  Out6 : Outport  Port=6
  wires:
  Vt/1 -> Add Watermark/1(y)
  It/1 -> Add Watermark1/1(y)
  Vout/1 -> Add Watermark2/1(y)
  Add Watermark/1(y_ym) -> Out2/1
  Add Watermark/2(wm) -> Out4/1
  Add Watermark1/1(y_ym) -> Out1/1
  Add Watermark1/2(wm) -> Out5/1
  Add Watermark2/1(y_ym) -> Out3/1
  Add Watermark2/2(wm) -> Out6/1

== system cyberAttack2/Communication Channel DGU 1 (open to attack)/Communication Channel ==
  Vt : Inport
  It : Inport  Port=2
  Vout : Inport  Port=3
  tag scope: It_1=global, Vout_1=global, Vt_1=global
  wires:
  Vout/1 -> [Vout_1]
  It/1 -> [It_1]
  Vt/1 -> [Vt_1]

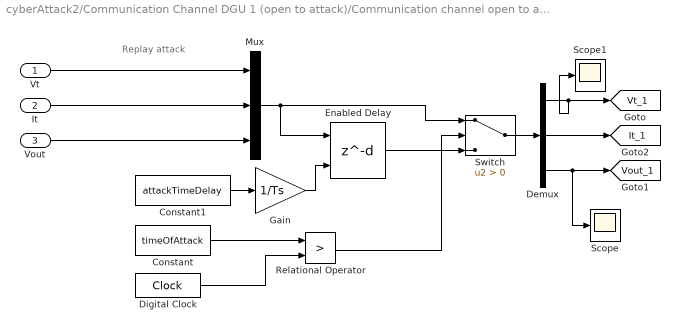
== system cyberAttack2/Communication Channel DGU 1 (open to attack)/Communication channel open to attack ==
  note: Replay attack
  Vt : Inport
  It : Inport  Port=2
  Vout : Inport  Port=3
  Constant : Constant  Value=timeOfAttack  SampleTime=1
  Constant1 : Constant  Value=attackTimeDelay
  Demux : Demux  Outputs=3
  Digital Clock : DigitalClock
  Enabled Delay : Delay  DelayLengthSource=Input port  DelayLength=attackTimeDelay/Ts  DelayLengthUpperLimit=4000  SampleTime=Ts
      settings: InputPortMap=u0,p1
  Gain : Gain  Gain=1/Ts
  Mux : Mux  Inputs=3
  Relational Operator : RelationalOperator  Operator=>  OutDataTypeStr=boolean  RndMeth=Simplest  InputSameDT=off
  Scope : Scope
  Scope1 : Scope
  Switch : Switch  Criteria=u2 > Threshold  SaturateOnIntegerOverflow=off  InputSameDT=off
  tag scope: It_1=global, Vout_1=global, Vt_1=global
  wires:
  Demux/1 -> Scope1/1, [Vt_1]
  Demux/2 -> [It_1]
  Demux/3 -> Scope/1, [Vout_1]
  Vout/1 -> Mux/3
  It/1 -> Mux/2
  Vt/1 -> Mux/1
  Constant1/1 -> Gain/1
  Constant/1 -> Relational Operator/1
  Switch/1 -> Demux/1
  Mux/1 -> Switch/1, Enabled Delay/1
  Relational Operator/1 -> Switch/2
  Enabled Delay/1 -> Switch/3
  Digital Clock/1 -> Relational Operator/2
  Gain/1 -> Enabled Delay/2

== system cyberAttack2/Communication Channel DGU 1 (open to attack)3/Communication Channel ==
  Vt : Inport
  It : Inport  Port=2
  Vout : Inport  Port=3
  tag scope: It_3=global, Vout_3=global, Vt_3=global
  wires:
  Vout/1 -> [Vout_3]
  It/1 -> [It_3]
  Vt/1 -> [Vt_3]
